simulink library "POSTPROC"  (Simulink 9.0)
settings: Solver=VariableStepAuto  StartTime=0.0  StopTime=10.0  RelTol=1e-3
undefined symbols (not defined in the file or in its folder): DYN_SC_par, SEN_GYR_par, SEN_MTM_par, SEN_SOL_par, SEN_SSS_par, sim_par
libraries: LIB_ROT x24, LIB_ORB x1
settings Model: Creator=alger  LastModifiedBy=alger

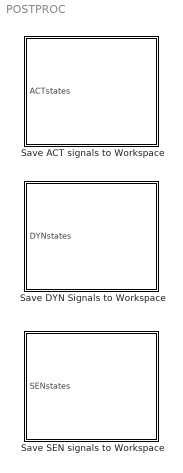
== system POSTPROC ==
  Save ACT signals to Workspace : Subsystem
  Save DYN Signals to Workspace : Subsystem
  Save SEN signals to Workspace : Subsystem

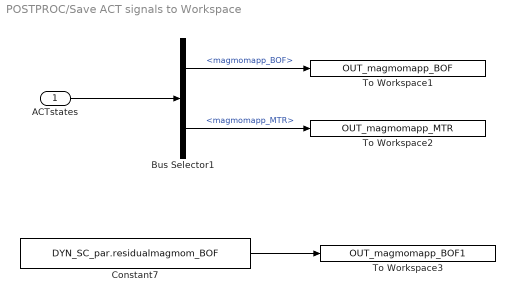
== system POSTPROC/Save ACT signals to Workspace ==
  ACTstates : Inport  SampleTime=sim_par.t_sample
  Bus Selector1 : BusSelector  OutputSignals=magmomapp_BOF,magmomapp_MTR
  Constant7 : Constant  Value=DYN_SC_par.residualmagmom_BOF
  To Workspace1 : ToWorkspace  VariableName=OUT_magmomapp_BOF  SaveFormat=Structure With Time  SampleTime=sim_par.t_sample
  To Workspace2 : ToWorkspace  VariableName=OUT_magmomapp_MTR  SaveFormat=Structure With Time  SampleTime=sim_par.t_sample
  To Workspace3 : ToWorkspace  VariableName=OUT_magmomapp_BOF1  SaveFormat=Structure With Time  SampleTime=sim_par.t_sample
  wires:
  Bus Selector1/2 -> To Workspace2/1  "<magmomapp_MTR>"
  Bus Selector1/1 -> To Workspace1/1  "<magmomapp_BOF>"
  ACTstates/1 -> Bus Selector1/1
  Constant7/1 -> To Workspace3/1

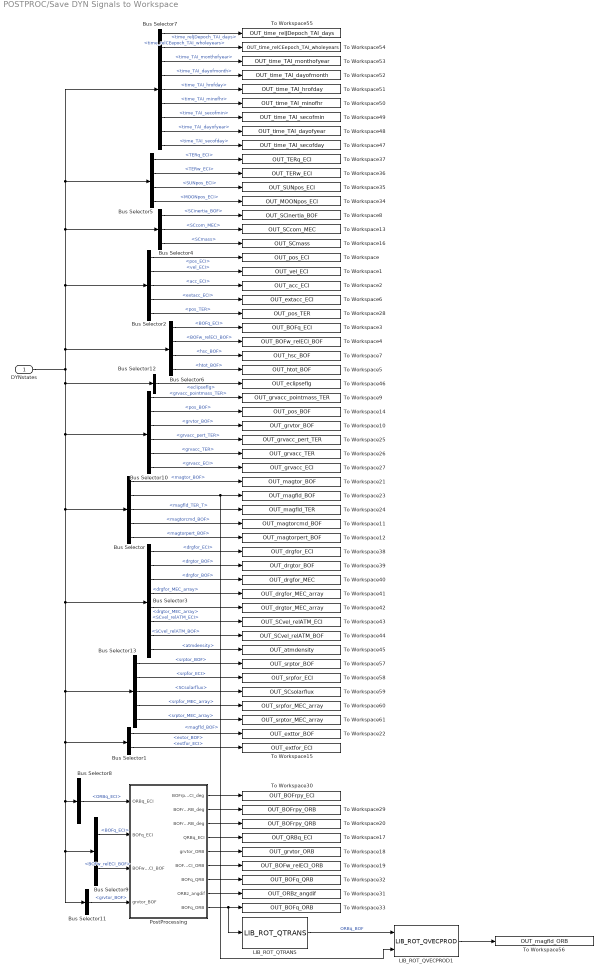
== system POSTPROC/Save DYN Signals to Workspace ==
  DYNstates : Inport  SampleTime=sim_par.t_sample
  Bus Selector : BusSelector  OutputSignals=magtor_BOF,magfld_BOF,magfld_TER_T,magtorcmd_BOF,magtorpert_BOF
  Bus Selector1 : BusSelector  OutputSignals=extor_BOF,extfor_ECI
  Bus Selector10 : BusSelector  OutputSignals=grvacc_pointmass_TER,pos_BOF,grvtor_BOF,grvacc_pert_TER,grvacc_TER,grvacc_ECI
  Bus Selector11 : BusSelector  OutputSignals=grvtor_BOF
  Bus Selector12 : BusSelector  OutputSignals=eclipseflg
  Bus Selector13 : BusSelector  OutputSignals=srptor_BOF,srpfor_ECI,SCsolarflux,srpfor_MEC_array,srptor_MEC_array
  Bus Selector2 : BusSelector  OutputSignals=pos_ECI,vel_ECI,acc_ECI,extacc_ECI,pos_TER
  Bus Selector3 : BusSelector  OutputSignals=drgfor_ECI,drgtor_BOF,drgfor_BOF,drgfor_MEC_array,drgtor_MEC_array,SCvel_relATM_ECI,SCvel_relATM_BOF,atmdensity
  Bus Selector4 : BusSelector  OutputSignals=SCinertia_BOF,SCcom_MEC,SCmass
  Bus Selector5 : BusSelector  OutputSignals=TERq_ECI,TERw_ECI,SUNpos_ECI,MOONpos_ECI
  Bus Selector6 : BusSelector  OutputSignals=BOFq_ECI,BOFw_relECI_BOF,hsc_BOF,htot_BOF
  Bus Selector7 : BusSelector  OutputSignals=time_relJDepoch_TAI_days,time_relCEepoch_TAI_wholeyears,time_TAI_monthofyear,time_TAI_dayofmonth,time_TAI_hrofday,time_TAI_minofhr,time_TAI_secofmin,time_TAI_dayofyear,time_TAI_secofday
  Bus Selector8 : BusSelector  OutputSignals=ORBq_ECI
  Bus Selector9 : BusSelector  OutputSignals=BOFq_ECI,BOFw_relECI_BOF
  LIB_ROT_QTRANS : LIB_ROT/LIB_ROT_QTRANS
  LIB_ROT_QVECPROD1 : LIB_ROT/LIB_ROT_QVECPROD
  PostProcessing : Subsystem
  To Workspace : ToWorkspace  VariableName=OUT_pos_ECI  SaveFormat=Structure With Time  SampleTime=sim_par.t_sample
  To Workspace1 : ToWorkspace  VariableName=OUT_vel_ECI  SaveFormat=Structure With Time  SampleTime=sim_par.t_sample
  To Workspace10 : ToWorkspace  VariableName=OUT_grvtor_BOF  SaveFormat=Structure With Time  SampleTime=sim_par.t_sample
  To Workspace11 : ToWorkspace  VariableName=OUT_magtorcmd_BOF  SaveFormat=Structure With Time  SampleTime=sim_par.t_sample
  To Workspace12 : ToWorkspace  VariableName=OUT_magtorpert_BOF  SaveFormat=Structure With Time  SampleTime=sim_par.t_sample
  To Workspace13 : ToWorkspace  VariableName=OUT_SCcom_MEC  SaveFormat=Structure With Time  SampleTime=sim_par.t_sample
  To Workspace14 : ToWorkspace  VariableName=OUT_pos_BOF  SaveFormat=Structure With Time  SampleTime=sim_par.t_sample
  To Workspace15 : ToWorkspace  VariableName=OUT_extfor_ECI  SaveFormat=Structure With Time  SampleTime=sim_par.t_sample
  To Workspace16 : ToWorkspace  VariableName=OUT_SCmass  SaveFormat=Structure With Time  SampleTime=sim_par.t_sample
  To Workspace17 : ToWorkspace  VariableName=OUT_QRBq_ECI  SaveFormat=Structure With Time  SampleTime=sim_par.t_sample
  To Workspace18 : ToWorkspace  VariableName=OUT_grvtor_ORB  SaveFormat=Structure With Time  SampleTime=sim_par.t_sample
  To Workspace19 : ToWorkspace  VariableName=OUT_BOFw_relECI_ORB  SaveFormat=Structure With Time  SampleTime=sim_par.t_sample
  To Workspace2 : ToWorkspace  VariableName=OUT_acc_ECI  SaveFormat=Structure With Time  SampleTime=sim_par.t_sample
  To Workspace20 : ToWorkspace  VariableName=OUT_BOFrpy_QRB  SaveFormat=Structure With Time  SampleTime=sim_par.t_sample
  To Workspace21 : ToWorkspace  VariableName=OUT_magtor_BOF  SaveFormat=Structure With Time  SampleTime=sim_par.t_sample
  To Workspace22 : ToWorkspace  VariableName=OUT_exttor_BOF  SaveFormat=Structure With Time  SampleTime=sim_par.t_sample
  To Workspace23 : ToWorkspace  VariableName=OUT_magfld_BOF  SaveFormat=Structure With Time  SampleTime=sim_par.t_sample
  To Workspace24 : ToWorkspace  VariableName=OUT_magfld_TER  SaveFormat=Structure With Time  SampleTime=sim_par.t_sample
  To Workspace25 : ToWorkspace  VariableName=OUT_grvacc_pert_TER  SaveFormat=Structure With Time  SampleTime=sim_par.t_sample
  To Workspace26 : ToWorkspace  VariableName=OUT_grvacc_TER  SaveFormat=Structure With Time  SampleTime=sim_par.t_sample
  To Workspace27 : ToWorkspace  VariableName=OUT_grvacc_ECI  SaveFormat=Structure With Time  SampleTime=sim_par.t_sample
  To Workspace28 : ToWorkspace  VariableName=OUT_pos_TER  SaveFormat=Structure With Time  SampleTime=sim_par.t_sample
  To Workspace29 : ToWorkspace  VariableName=OUT_BOFrpy_ORB  SaveFormat=Structure With Time  SampleTime=sim_par.t_sample
  To Workspace3 : ToWorkspace  VariableName=OUT_BOFq_ECI  SaveFormat=Structure With Time  SampleTime=sim_par.t_sample
  To Workspace30 : ToWorkspace  VariableName=OUT_BOFrpy_ECI  SaveFormat=Structure With Time  SampleTime=sim_par.t_sample
  To Workspace31 : ToWorkspace  VariableName=OUT_ORBz_angdif  SaveFormat=Structure With Time  SampleTime=sim_par.t_sample
  To Workspace32 : ToWorkspace  VariableName=OUT_BOFq_QRB  SaveFormat=Structure With Time  SampleTime=sim_par.t_sample
  To Workspace33 : ToWorkspace  VariableName=OUT_BOFq_ORB  SaveFormat=Structure With Time  SampleTime=sim_par.t_sample
  To Workspace34 : ToWorkspace  VariableName=OUT_MOONpos_ECI  SaveFormat=Structure With Time  SampleTime=sim_par.t_sample
  To Workspace35 : ToWorkspace  VariableName=OUT_SUNpos_ECI  SaveFormat=Structure With Time  SampleTime=sim_par.t_sample
  To Workspace36 : ToWorkspace  VariableName=OUT_TERw_ECI  SaveFormat=Structure With Time  SampleTime=sim_par.t_sample
  To Workspace37 : ToWorkspace  VariableName=OUT_TERq_ECI  SaveFormat=Structure With Time  SampleTime=sim_par.t_sample
  To Workspace38 : ToWorkspace  VariableName=OUT_drgfor_ECI  SaveFormat=Structure With Time  SampleTime=sim_par.t_sample
  To Workspace39 : ToWorkspace  VariableName=OUT_drgtor_BOF  SaveFormat=Structure With Time  SampleTime=sim_par.t_sample
  To Workspace4 : ToWorkspace  VariableName=OUT_BOFw_relECI_BOF  SaveFormat=Structure With Time  SampleTime=sim_par.t_sample
  To Workspace40 : ToWorkspace  VariableName=OUT_drgfor_MEC  SaveFormat=Structure With Time  SampleTime=sim_par.t_sample
  To Workspace41 : ToWorkspace  VariableName=OUT_drgfor_MEC_array  SaveFormat=Structure With Time  SampleTime=sim_par.t_sample
  To Workspace42 : ToWorkspace  VariableName=OUT_drgtor_MEC_array  SaveFormat=Structure With Time  SampleTime=sim_par.t_sample
  To Workspace43 : ToWorkspace  VariableName=OUT_SCvel_relATM_ECI  SaveFormat=Structure With Time  SampleTime=sim_par.t_sample
  To Workspace44 : ToWorkspace  VariableName=OUT_SCvel_relATM_BOF  SaveFormat=Structure With Time  SampleTime=sim_par.t_sample
  To Workspace45 : ToWorkspace  VariableName=OUT_atmdensity  SaveFormat=Structure With Time  SampleTime=sim_par.t_sample
  To Workspace46 : ToWorkspace  VariableName=OUT_eclipseflg  SaveFormat=Structure With Time  SampleTime=sim_par.t_sample
  To Workspace47 : ToWorkspace  VariableName=OUT_time_TAI_secofday  SaveFormat=Structure With Time  SampleTime=sim_par.t_sample
  To Workspace48 : ToWorkspace  VariableName=OUT_time_TAI_dayofyear  SaveFormat=Structure With Time  SampleTime=sim_par.t_sample
  To Workspace49 : ToWorkspace  VariableName=OUT_time_TAI_secofmin  SaveFormat=Structure With Time  SampleTime=sim_par.t_sample
  To Workspace5 : ToWorkspace  VariableName=OUT_htot_BOF  SaveFormat=Structure With Time  SampleTime=sim_par.t_sample
  To Workspace50 : ToWorkspace  VariableName=OUT_time_TAI_minofhr  SaveFormat=Structure With Time  SampleTime=sim_par.t_sample
  To Workspace51 : ToWorkspace  VariableName=OUT_time_TAI_hrofday  SaveFormat=Structure With Time  SampleTime=sim_par.t_sample
  To Workspace52 : ToWorkspace  VariableName=OUT_time_TAI_dayofmonth  SaveFormat=Structure With Time  SampleTime=sim_par.t_sample
  To Workspace53 : ToWorkspace  VariableName=OUT_time_TAI_monthofyear  SaveFormat=Structure With Time  SampleTime=sim_par.t_sample
  To Workspace54 : ToWorkspace  VariableName=OUT_time_relCEepoch_TAI_wholeyears  SaveFormat=Structure With Time  SampleTime=sim_par.t_sample
  To Workspace55 : ToWorkspace  VariableName=OUT_time_relJDepoch_TAI_days  SaveFormat=Structure With Time  SampleTime=sim_par.t_sample
  To Workspace56 : ToWorkspace  VariableName=OUT_magfld_ORB  SaveFormat=Structure With Time  SampleTime=sim_par.t_sample
  To Workspace57 : ToWorkspace  VariableName=OUT_srptor_BOF  SaveFormat=Structure With Time  SampleTime=sim_par.t_sample
  To Workspace58 : ToWorkspace  VariableName=OUT_srpfor_ECI  SaveFormat=Structure With Time  SampleTime=sim_par.t_sample
  To Workspace59 : ToWorkspace  VariableName=OUT_SCsolarflux  SaveFormat=Structure With Time  SampleTime=sim_par.t_sample
  To Workspace6 : ToWorkspace  VariableName=OUT_extacc_ECI  SaveFormat=Structure With Time  SampleTime=sim_par.t_sample
  To Workspace60 : ToWorkspace  VariableName=OUT_srpfor_MEC_array  SaveFormat=Structure With Time  SampleTime=sim_par.t_sample
  To Workspace61 : ToWorkspace  VariableName=OUT_srptor_MEC_array  SaveFormat=Structure With Time  SampleTime=sim_par.t_sample
  To Workspace7 : ToWorkspace  VariableName=OUT_hsc_BOF  SaveFormat=Structure With Time  SampleTime=sim_par.t_sample
  To Workspace8 : ToWorkspace  VariableName=OUT_SCinertia_BOF  SaveFormat=Structure With Time  SampleTime=sim_par.t_sample
  To Workspace9 : ToWorkspace  VariableName=OUT_grvacc_pointmass_TER  SaveFormat=Structure With Time  SampleTime=sim_par.t_sample
  wires:
  Bus Selector13/5 -> To Workspace61/1  "<srptor_MEC_array>"
  Bus Selector13/4 -> To Workspace60/1  "<srpfor_MEC_array>"
  Bus Selector13/3 -> To Workspace59/1  "<SCsolarflux>"
  Bus Selector13/2 -> To Workspace58/1  "<srpfor_ECI>"
  Bus Selector13/1 -> To Workspace57/1  "<srptor_BOF>"
  LIB_ROT_QVECPROD1/1 -> To Workspace56/1
  LIB_ROT_QTRANS/1 -> LIB_ROT_QVECPROD1/1  "ORBq_BOF"
  Bus Selector/2 -> LIB_ROT_QVECPROD1/2, To Workspace23/1  "<magfld_BOF>"
  Bus Selector10/2 -> To Workspace14/1  "<pos_BOF>"
  Bus Selector6/4 -> To Workspace5/1  "<htot_BOF>"
  Bus Selector2/3 -> To Workspace2/1  "<acc_ECI>"
  Bus Selector4/3 -> To Workspace16/1  "<SCmass>"
  Bus Selector5/4 -> To Workspace34/1  "<MOONpos_ECI>"
  Bus Selector6/1 -> To Workspace3/1  "<BOFq_ECI>"
  Bus Selector2/5 -> To Workspace28/1  "<pos_TER>"
  Bus Selector2/2 -> To Workspace1/1  "<vel_ECI>"
  Bus Selector5/2 -> To Workspace36/1  "<TERw_ECI>"
  Bus Selector3/2 -> To Workspace39/1  "<drgtor_BOF>"
  Bus Selector3/3 -> To Workspace40/1  "<drgfor_BOF>"
  Bus Selector4/2 -> To Workspace13/1  "<SCcom_MEC>"
  Bus Selector4/1 -> To Workspace8/1  "<SCinertia_BOF>"
  Bus Selector3/4 -> To Workspace41/1  "<drgfor_MEC_array>"
  Bus Selector3/5 -> To Workspace42/1  "<drgtor_MEC_array>"
  Bus Selector/5 -> To Workspace12/1  "<magtorpert_BOF>"
  Bus Selector/4 -> To Workspace11/1  "<magtorcmd_BOF>"
  Bus Selector2/4 -> To Workspace6/1  "<extacc_ECI>"
  Bus Selector/3 -> To Workspace24/1  "<magfld_TER_T>"
  Bus Selector6/3 -> To Workspace7/1  "<hsc_BOF>"
  Bus Selector6/2 -> To Workspace4/1  "<BOFw_relECI_BOF>"
  Bus Selector5/3 -> To Workspace35/1  "<SUNpos_ECI>"
  Bus Selector10/4 -> To Workspace25/1  "<grvacc_pert_TER>"
  Bus Selector2/1 -> To Workspace/1  "<pos_ECI>"
  Bus Selector10/3 -> To Workspace10/1  "<grvtor_BOF>"
  Bus Selector/1 -> To Workspace21/1  "<magtor_BOF>"
  Bus Selector10/6 -> To Workspace27/1  "<grvacc_ECI>"
  Bus Selector10/1 -> To Workspace9/1  "<grvacc_pointmass_TER>"
  Bus Selector10/5 -> To Workspace26/1  "<grvacc_TER>"
  Bus Selector5/1 -> To Workspace37/1  "<TERq_ECI>"
  PostProcessing/9(BOFq_ORB) -> To Workspace33/1, LIB_ROT_QTRANS/1
  Bus Selector12/1 -> To Workspace46/1  "<eclipseflg>"
  Bus Selector9/1 -> PostProcessing/2(BOFq_ECI)  "<BOFq_ECI>"
  PostProcessing/5(grvtor_ORB) -> To Workspace18/1
  Bus Selector9/2 -> PostProcessing/3(BOFw_relECI_BOF)  "<BOFw_relECI_BOF>"
  PostProcessing/6(BOFw_relECI_ORB) -> To Workspace19/1
  PostProcessing/4(QRBq_ECI) -> To Workspace17/1
  Bus Selector1/2 -> To Workspace15/1  "<extfor_ECI>"
  Bus Selector3/1 -> To Workspace38/1  "<drgfor_ECI>"
  Bus Selector7/3 -> To Workspace53/1  "<time_TAI_monthofyear>"
  PostProcessing/1(BOFrpy_ECI_deg) -> To Workspace30/1
  Bus Selector7/1 -> To Workspace55/1  "<time_relJDepoch_TAI_days>"
  PostProcessing/7(BOFq_QRB) -> To Workspace32/1
  Bus Selector7/9 -> To Workspace47/1  "<time_TAI_secofday>"
  Bus Selector7/8 -> To Workspace48/1  "<time_TAI_dayofyear>"
  PostProcessing/8(ORBz_angdif) -> To Workspace31/1
  Bus Selector7/2 -> To Workspace54/1  "<time_relCEepoch_TAI_wholeyears>"
  Bus Selector7/7 -> To Workspace49/1  "<time_TAI_secofmin>"
  Bus Selector7/5 -> To Workspace51/1  "<time_TAI_hrofday>"
  Bus Selector7/6 -> To Workspace50/1  "<time_TAI_minofhr>"
  Bus Selector7/4 -> To Workspace52/1  "<time_TAI_dayofmonth>"
  DYNstates/1 -> Bus Selector2/1, Bus Selector7/1, Bus Selector5/1, Bus Selector4/1, Bus Selector6/1, Bus Selector10/1, Bus Selector/1, Bus Selector3/1, Bus Selector13/1, Bus Selector1/1, Bus Selector8/1, Bus Selector9/1, Bus Selector11/1, Bus Selector12/1
  PostProcessing/2(BOFrpy_ORB_deg) -> To Workspace29/1
  PostProcessing/3(BOFrpy_QRB_deg) -> To Workspace20/1
  Bus Selector8/1 -> PostProcessing/1(ORBq_ECI)  "<ORBq_ECI>"
  Bus Selector11/1 -> PostProcessing/4(grvtor_BOF)  "<grvtor_BOF>"
  Bus Selector3/6 -> To Workspace43/1  "<SCvel_relATM_ECI>"
  Bus Selector3/8 -> To Workspace45/1  "<atmdensity>"
  Bus Selector3/7 -> To Workspace44/1  "<SCvel_relATM_BOF>"
  Bus Selector1/1 -> To Workspace22/1  "<extor_BOF>"

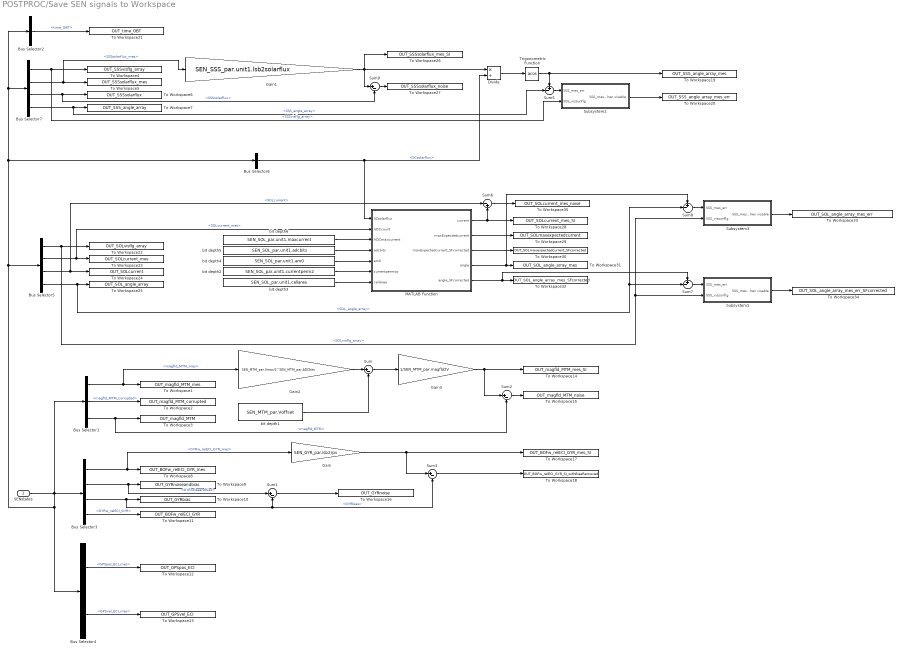
== system POSTPROC/Save SEN signals to Workspace ==
  SENstates : Inport  SampleTime=sim_par.t_sample
  Bus Selector1 : BusSelector  OutputSignals=magfld_MTM_mes,magfld_MTM_corrupted,magfld_MTM
  Bus Selector2 : BusSelector  OutputSignals=time_OBT
  Bus Selector3 : BusSelector  OutputSignals=GYRw_relECI_GYR_mes,GYRnoiseandbias,GYRbias,GYRw_relECI_GYR
  Bus Selector4 : BusSelector  OutputSignals=GPSpos_ECI_mes,GPSvel_ECI_mes
  Bus Selector5 : BusSelector  OutputSignals=SOLvisflg_array,SOLcurrent_mes,SOLcurrent,SOL_angle_array
  Bus Selector6 : BusSelector  OutputSignals=SCsolarflux
  Bus Selector7 : BusSelector  OutputSignals=SSSvisflg_array,SSSsolarflux_mes,SSSsolarflux,SSS_angle_array
  Divide : Product  Inputs=*/
  Gain : Gain  Gain=SEN_GYR_par.lsb2rps
  Gain1 : Gain  Gain=SEN_SSS_par.unit1.lsb2solarflux
  Gain2 : Gain  Gain=SEN_MTM_par.Vmax/2^SEN_MTM_par.ADCbits
  Gain3 : Gain  Gain=1/SEN_MTM_par.magfld2V
  MATLAB Function : MATLAB Function  TreatAsAtomicUnit=on
  Subsystem1 : Subsystem
  Subsystem2 : Subsystem
  Subsystem3 : Subsystem
  Sum{,1..3,9} (5 alike) : Sum  Inputs=|+-
  Sum5 : Sum  Inputs=+-|
  Sum6 : Sum  Inputs=|-+
  Sum7 : Sum  Inputs=+-|
  Sum8 : Sum  Inputs=+-|
  To Workspace1 : ToWorkspace  VariableName=OUT_magfld_MTM_mes  SaveFormat=Structure With Time  SampleTime=sim_par.t_sample
  To Workspace10 : ToWorkspace  VariableName=OUT_GYRbias  SaveFormat=Structure With Time  SampleTime=sim_par.t_sample
  To Workspace11 : ToWorkspace  VariableName=OUT_BOFw_relECI_GYR  SaveFormat=Structure With Time  SampleTime=sim_par.t_sample
  To Workspace12 : ToWorkspace  VariableName=OUT_GPSpos_ECI  SaveFormat=Structure With Time  SampleTime=sim_par.t_sample
  To Workspace13 : ToWorkspace  VariableName=OUT_GPSvel_ECI  SaveFormat=Structure With Time  SampleTime=sim_par.t_sample
  To Workspace14 : ToWorkspace  VariableName=OUT_magfld_MTM_mes_SI  SaveFormat=Structure With Time  SampleTime=sim_par.t_sample
  To Workspace15 : ToWorkspace  VariableName=OUT_magfld_MTM_noise  SaveFormat=Structure With Time  SampleTime=sim_par.t_sample
  To Workspace16 : ToWorkspace  VariableName=OUT_GYRnoise  SaveFormat=Structure With Time  SampleTime=sim_par.t_sample
  To Workspace17 : ToWorkspace  VariableName=OUT_BOFw_relECI_GYR_mes_SI  SaveFormat=Structure With Time  SampleTime=sim_par.t_sample
  To Workspace18 : ToWorkspace  VariableName=OUT_BOFw_relECI_GYR_SI_withBiasRemoved  SaveFormat=Structure With Time  SampleTime=sim_par.t_sample
  To Workspace19 : ToWorkspace  VariableName=OUT_SSS_angle_array_mes  SaveFormat=Structure With Time  SampleTime=sim_par.t_sample
  To Workspace2 : ToWorkspace  VariableName=OUT_magfld_MTM_corrupted  SaveFormat=Structure With Time  SampleTime=sim_par.t_sample
  To Workspace20 : ToWorkspace  VariableName=OUT_SSS_angle_array_mes_err  SaveFormat=Structure With Time  SampleTime=sim_par.t_sample
  To Workspace21 : ToWorkspace  VariableName=OUT_time_OBT  SaveFormat=Structure With Time  SampleTime=sim_par.t_sample
  To Workspace22 : ToWorkspace  VariableName=OUT_SOLvisflg_array  SaveFormat=Structure With Time  SampleTime=sim_par.t_sample
  To Workspace23 : ToWorkspace  VariableName=OUT_SOLcurrent_mes  SaveFormat=Structure With Time  SampleTime=sim_par.t_sample
  To Workspace24 : ToWorkspace  VariableName=OUT_SOLcurrent  SaveFormat=Structure With Time  SampleTime=sim_par.t_sample
  To Workspace25 : ToWorkspace  VariableName=OUT_SOL_angle_array  SaveFormat=Structure With Time  SampleTime=sim_par.t_sample
  To Workspace26 : ToWorkspace  VariableName=OUT_SSSsolarflux_mes_SI  SaveFormat=Structure With Time  SampleTime=sim_par.t_sample
  To Workspace27 : ToWorkspace  VariableName=OUT_SSSsolarflux_noise  SaveFormat=Structure With Time  SampleTime=sim_par.t_sample
  To Workspace28 : ToWorkspace  VariableName=OUT_SOLcurrent_mes_SI  SaveFormat=Structure With Time  SampleTime=sim_par.t_sample
  To Workspace29 : ToWorkspace  VariableName=OUT_SOLmaxexpectedcurrent  SaveFormat=Structure With Time  SampleTime=sim_par.t_sample
  To Workspace3 : ToWorkspace  VariableName=OUT_magfld_MTM  SaveFormat=Structure With Time  SampleTime=sim_par.t_sample
  To Workspace30 : ToWorkspace  VariableName=OUT_SOLmaxexpectedcurrent_SFcorrected  SaveFormat=Structure With Time  SampleTime=sim_par.t_sample
  To Workspace31 : ToWorkspace  VariableName=OUT_SOL_angle_array_mes  SaveFormat=Structure With Time  SampleTime=sim_par.t_sample
  To Workspace32 : ToWorkspace  VariableName=OUT_SOL_angle_array_mes_SFcorrected  SaveFormat=Structure With Time  SampleTime=sim_par.t_sample
  To Workspace33 : ToWorkspace  VariableName=OUT_SOL_angle_array_mes_err  SaveFormat=Structure With Time  SampleTime=sim_par.t_sample
  To Workspace34 : ToWorkspace  VariableName=OUT_SOL_angle_array_mes_err_SFcorrected  SaveFormat=Structure With Time  SampleTime=sim_par.t_sample
  To Workspace35 : ToWorkspace  VariableName=OUT_SOLcurrent_mes_noise  SaveFormat=Structure With Time  SampleTime=sim_par.t_sample
  To Workspace4 : ToWorkspace  VariableName=OUT_SSSvisflg_array  SaveFormat=Structure With Time  SampleTime=sim_par.t_sample
  To Workspace5 : ToWorkspace  VariableName=OUT_SSSsolarflux_mes  SaveFormat=Structure With Time  SampleTime=sim_par.t_sample
  To Workspace6 : ToWorkspace  VariableName=OUT_SSSsolarflux  SaveFormat=Structure With Time  SampleTime=sim_par.t_sample
  To Workspace7 : ToWorkspace  VariableName=OUT_SSS_angle_array  SaveFormat=Structure With Time  SampleTime=sim_par.t_sample
  To Workspace8 : ToWorkspace  VariableName=OUT_BOFw_relECI_GYR_mes  SaveFormat=Structure With Time  SampleTime=sim_par.t_sample
  To Workspace9 : ToWorkspace  VariableName=OUT_GYRnoiseandbias  SaveFormat=Structure With Time  SampleTime=sim_par.t_sample
  Trigonometric Function : Trigonometry  Operator=acos  OutputSignalType=real
  bit depth1 : Constant  Value=SEN_MTM_par.Voffset
  bit depth2 : Constant  Value=SEN_SOL_par.unit1.currentperm2
  bit depth3 : Constant  Value=SEN_SOL_par.unit1.cellarea
  bit depth4 : Constant  Value=SEN_SOL_par.unit1.am0
  bit depth5 : Constant  Value=SEN_SOL_par.unit1.adcbits
  bit depth6 : Constant  Value=SEN_SOL_par.unit1.maxcurrent
  wires:
  MATLAB Function/3(maxExpectedcurrent_SFcorrected) -> To Workspace30/1
  Sum9/1 -> To Workspace27/1
  Divide/1 -> Trigonometric Function/1
  MATLAB Function/2(maxExpectedcurrent) -> To Workspace29/1
  Subsystem3/1(SSS_mes_err when visable) -> To Workspace33/1
  Sum8/1 -> Subsystem3/1(SSS_mes_err)
  MATLAB Function/4(angle) -> Sum8/1, To Workspace31/1
  Bus Selector5/4 -> To Workspace25/1, Sum8/2, Sum7/2  "<SOL_angle_array>"
  Bus Selector5/1 -> To Workspace22/1, Subsystem3/2(SSS_vissunflg), Subsystem1/2(SSS_vissunflg)  "<SOLvisflg_array>"
  Subsystem1/1(SSS_mes_err when visable) -> To Workspace34/1
  Sum7/1 -> Subsystem1/1(SSS_mes_err)
  MATLAB Function/5(angle_SFcorrected) -> To Workspace32/1, Sum7/1
  Sum6/1 -> To Workspace35/1
  bit depth6/1 -> MATLAB Function/3(ADCmaxcurrent)
  bit depth5/1 -> MATLAB Function/4(adcbits)
  bit depth4/1 -> MATLAB Function/5(am0)
  bit depth3/1 -> MATLAB Function/7(cellarea)
  bit depth2/1 -> MATLAB Function/6(currentpermsq)
  MATLAB Function/1(current) -> Sum6/2, To Workspace28/1
  Bus Selector6/1 -> MATLAB Function/1(SCsolarflux), Divide/2  "<SCsolarflux>"
  Bus Selector5/3 -> To Workspace24/1, Sum6/1  "<SOLcurrent>"
  Bus Selector5/2 -> To Workspace23/1, MATLAB Function/2(ADCcount)  "<SOLcurrent_mes>"
  Bus Selector2/1 -> To Workspace21/1  "<time_OBT>"
  SENstates/1 -> Bus Selector5/1, Bus Selector6/1, Bus Selector7/1, Bus Selector2/1, Bus Selector4/1, Bus Selector1/1, Bus Selector3/1
  Bus Selector1/1 -> Gain2/1, To Workspace1/1  "<magfld_MTM_mes>"
  Bus Selector1/2 -> To Workspace2/1  "<magfld_MTM_corrupted>"
  Bus Selector1/3 -> Sum2/2, To Workspace3/1  "<magfld_MTM>"
  Bus Selector7/1 -> To Workspace4/1, Subsystem2/2(SSS_vissunflg)  "<SSSvisflg_array>"
  Bus Selector7/4 -> Sum5/2, To Workspace7/1  "<SSS_angle_array>"
  Bus Selector7/3 -> To Workspace6/1, Sum9/2  "<SSSsolarflux>"
  Bus Selector7/2 -> Gain1/1, To Workspace5/1  "<SSSsolarflux_mes>"
  Bus Selector3/1 -> Gain/1, To Workspace8/1  "<GYRw_relECI_GYR_mes>"
  Bus Selector3/2 -> Sum1/1, To Workspace9/1  "<GYRnoiseandbias>"
  Bus Selector3/3 -> Sum1/2, Sum3/2, To Workspace10/1  "<GYRbias>"
  Bus Selector3/4 -> To Workspace11/1  "<GYRw_relECI_GYR>"
  Bus Selector4/1 -> To Workspace12/1  "<GPSpos_ECI_mes>"
  Bus Selector4/2 -> To Workspace13/1  "<GPSvel_ECI_mes>"
  Sum/1 -> Gain3/1
  Gain2/1 -> Sum/1
  bit depth1/1 -> Sum/2
  Gain3/1 -> Sum2/1, To Workspace14/1
  Sum2/1 -> To Workspace15/1
  Sum1/1 -> To Workspace16/1
  Gain/1 -> Sum3/1, To Workspace17/1
  Sum3/1 -> To Workspace18/1
  Gain1/1 -> Sum9/1, Divide/1, To Workspace26/1
  Sum5/1 -> Subsystem2/1(SSS_mes_err)
  Trigonometric Function/1 -> To Workspace19/1, Sum5/1
  Subsystem2/1(SSS_mes_err when visable) -> To Workspace20/1

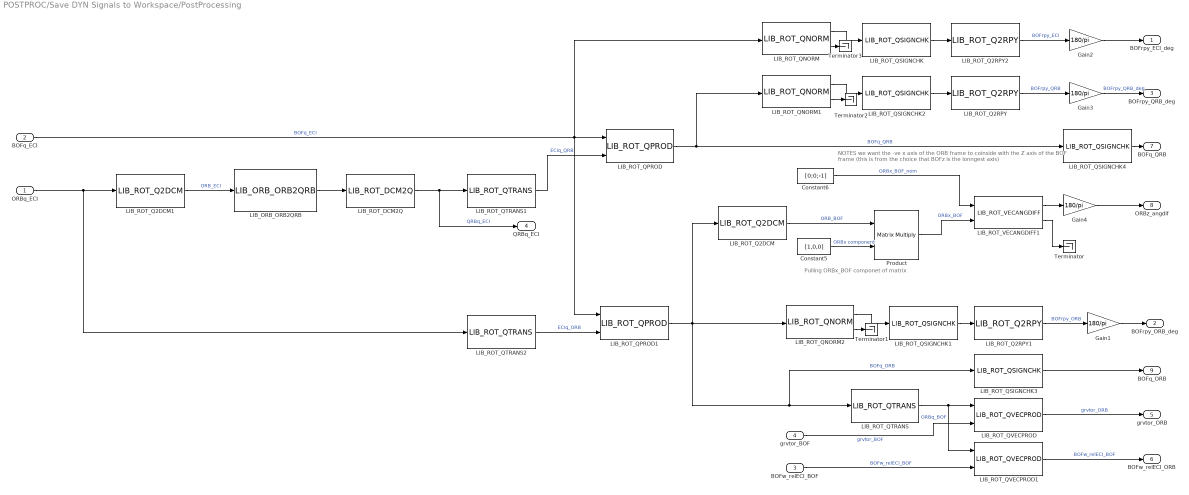
== system POSTPROC/Save DYN Signals to Workspace/PostProcessing ==
  note: Pulling ORBx_BOF componet of matrix
  note: NOTES
      | we want the -ve x axis of the ORB frame to coinside with the Z axis of the BOF frame
      | (this is from the choice that BOFz is the lonngest axis)
  ORBq_ECI : Inport
  BOFq_ECI : Inport  Port=2
  BOFw_relECI_BOF : Inport  Port=3
  grvtor_BOF : Inport  Port=4
  Constant5 : Constant  Value=[1,0,0]
  Constant6 : Constant  Value=[0;0;-1]
  Gain{1..4} (4 alike) : Gain  Gain=180/pi
  LIB_ORB_ORB2QRB : LIB_ORB/LIB_ORB_ORB2QRB
  LIB_ROT_DCM2Q : LIB_ROT/LIB_ROT_DCM2Q
  LIB_ROT_Q2DCM : LIB_ROT/LIB_ROT_Q2DCM
  LIB_ROT_Q2DCM1 : LIB_ROT/LIB_ROT_Q2DCM
  LIB_ROT_Q2RPY : LIB_ROT/LIB_ROT_Q2RPY
  LIB_ROT_Q2RPY1 : LIB_ROT/LIB_ROT_Q2RPY
  LIB_ROT_Q2RPY2 : LIB_ROT/LIB_ROT_Q2RPY
  LIB_ROT_QNORM : LIB_ROT/LIB_ROT_QNORM  zero_tol=0
  LIB_ROT_QNORM1 : LIB_ROT/LIB_ROT_QNORM  zero_tol=0
  LIB_ROT_QNORM2 : LIB_ROT/LIB_ROT_QNORM  zero_tol=0
  LIB_ROT_QPROD : LIB_ROT/LIB_ROT_QPROD
  LIB_ROT_QPROD1 : LIB_ROT/LIB_ROT_QPROD
  LIB_ROT_QSIGNCHK{,1..4} (5 alike) : LIB_ROT/LIB_ROT_QSIGNCHK
  LIB_ROT_QTRANS : LIB_ROT/LIB_ROT_QTRANS
  LIB_ROT_QTRANS1 : LIB_ROT/LIB_ROT_QTRANS
  LIB_ROT_QTRANS2 : LIB_ROT/LIB_ROT_QTRANS
  LIB_ROT_QVECPROD : LIB_ROT/LIB_ROT_QVECPROD
  LIB_ROT_QVECPROD1 : LIB_ROT/LIB_ROT_QVECPROD
  LIB_ROT_VECANGDIFF1 : LIB_ROT/LIB_ROT_VECANGDIFF  zero_tol=0
  Product : Product  Multiplication=Matrix(*)
  Terminator{,1..3} (4 alike) : Terminator
  BOFrpy_ECI_deg : Outport
  BOFrpy_ORB_deg : Outport  Port=2
  BOFrpy_QRB_deg : Outport  Port=3
  QRBq_ECI : Outport  Port=4
  grvtor_ORB : Outport  Port=5
  BOFw_relECI_ORB : Outport  Port=6
  BOFq_QRB : Outport  Port=7
  ORBz_angdif : Outport  Port=8
  BOFq_ORB : Outport  Port=9
  wires:
  LIB_ROT_QNORM/2 -> Terminator3/1
  LIB_ROT_QNORM1/2 -> Terminator2/1
  LIB_ROT_QNORM2/2 -> Terminator1/1
  LIB_ROT_QNORM/1 -> LIB_ROT_QSIGNCHK/1
  LIB_ROT_QNORM1/1 -> LIB_ROT_QSIGNCHK2/1
  LIB_ROT_QNORM2/1 -> LIB_ROT_QSIGNCHK1/1
  LIB_ROT_QSIGNCHK4/1 -> BOFq_QRB/1
  LIB_ROT_QSIGNCHK3/1 -> BOFq_ORB/1
  LIB_ROT_VECANGDIFF1/1 -> Gain4/1
  Gain4/1 -> ORBz_angdif/1
  LIB_ROT_QPROD1/1 -> LIB_ROT_Q2DCM/1, LIB_ROT_QNORM2/1, LIB_ROT_QTRANS/1, LIB_ROT_QSIGNCHK3/1  "BOFq_ORB"
  LIB_ROT_QTRANS/1 -> LIB_ROT_QVECPROD1/1, LIB_ROT_QVECPROD/1  "ORBq_BOF"
  LIB_ROT_QVECPROD/1 -> grvtor_ORB/1  "grvtor_ORB"
  LIB_ROT_QVECPROD1/1 -> BOFw_relECI_ORB/1  "BOFw_relECI_BOF"
  LIB_ROT_QSIGNCHK1/1 -> LIB_ROT_Q2RPY1/1
  LIB_ROT_Q2RPY1/1 -> Gain1/1  "BOFrpy_ORB"
  LIB_ROT_QSIGNCHK/1 -> LIB_ROT_Q2RPY2/1
  LIB_ROT_Q2RPY/1 -> Gain3/1  "BOFrpy_QRB"
  LIB_ROT_Q2RPY2/1 -> Gain2/1  "BOFrpy_ECI"
  LIB_ROT_QSIGNCHK2/1 -> LIB_ROT_Q2RPY/1
  LIB_ROT_Q2DCM/1 -> Product/1  "ORB_BOF"
  Constant6/1 -> LIB_ROT_VECANGDIFF1/1  "ORBx_BOF_nom"
  Constant5/1 -> Product/2  "ORBx component"
  Product/1 -> LIB_ROT_VECANGDIFF1/2  "ORBx_BOF"
  grvtor_BOF/1 -> LIB_ROT_QVECPROD/2  "grvtor_BOF"
  BOFw_relECI_BOF/1 -> LIB_ROT_QVECPROD1/2  "BOFw_relECI_BOF"
  LIB_ROT_VECANGDIFF1/2 -> Terminator/1
  Gain2/1 -> BOFrpy_ECI_deg/1
  Gain1/1 -> BOFrpy_ORB_deg/1
  Gain3/1 -> BOFrpy_QRB_deg/1  "BOFrpy_QRB_deg"
  BOFq_ECI/1 -> LIB_ROT_QPROD1/1, LIB_ROT_QPROD/1, LIB_ROT_QNORM/1  "BOFq_ECI"
  LIB_ORB_ORB2QRB/1 -> LIB_ROT_DCM2Q/1
  LIB_ROT_QPROD/1 -> LIB_ROT_QSIGNCHK4/1, LIB_ROT_QNORM1/1  "BOFq_QRB"
  LIB_ROT_DCM2Q/1 -> QRBq_ECI/1, LIB_ROT_QTRANS1/1  "QRBq_ECI"
  LIB_ROT_QTRANS1/1 -> LIB_ROT_QPROD/2  "ECIq_QRB"
  LIB_ROT_Q2DCM1/1 -> LIB_ORB_ORB2QRB/1  "ORB_ECI"
  LIB_ROT_QTRANS2/1 -> LIB_ROT_QPROD1/2  "ECIq_ORB"
  ORBq_ECI/1 -> LIB_ROT_Q2DCM1/1, LIB_ROT_QTRANS2/1

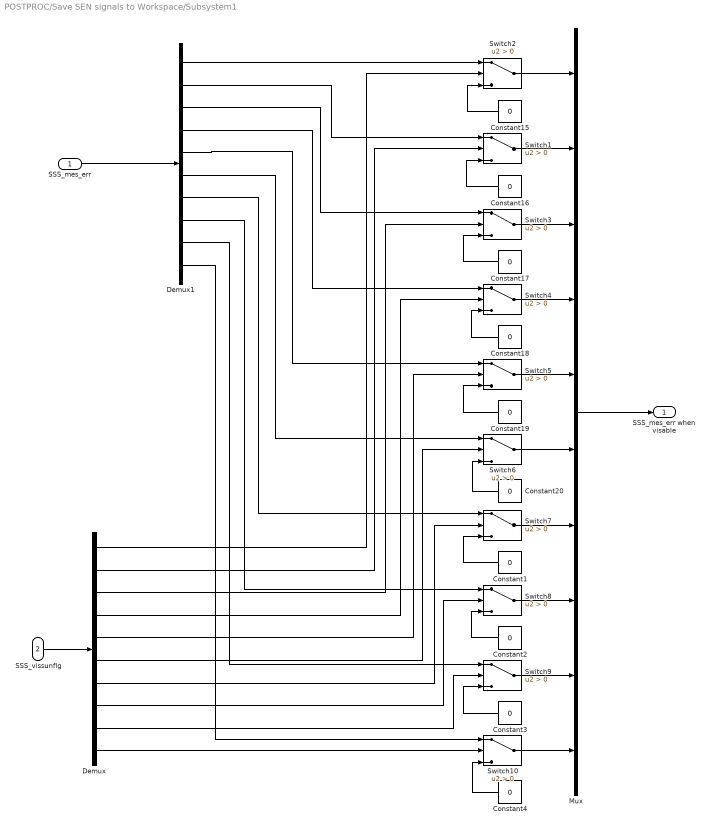
== system POSTPROC/Save SEN signals to Workspace/Subsystem1 ==
  SSS_mes_err : Inport
  SSS_vissunflg : Inport  Port=2
  Constant{1..4,15..20} (10 alike) : Constant  Value=0
  Demux : Demux  Outputs=10
  Demux1 : Demux  Outputs=10
  Mux : Mux  Inputs=10
  Switch{1..10} (10 alike) : Switch  Criteria=u2 > Threshold
  SSS_mes_err when visable : Outport
  wires:
  Demux1/8 -> Switch8/1
  Demux1/7 -> Switch7/1
  Constant4/1 -> Switch10/3
  Constant3/1 -> Switch9/3
  Demux/7 -> Switch7/2
  Switch10/1 -> Mux/10
  Demux/8 -> Switch8/2
  Demux1/9 -> Switch9/1
  Demux1/10 -> Switch10/1
  Constant1/1 -> Switch7/3
  Demux/9 -> Switch9/2
  Constant2/1 -> Switch8/3
  Switch7/1 -> Mux/7
  Switch9/1 -> Mux/9
  Demux/10 -> Switch10/2
  Switch8/1 -> Mux/8
  Constant20/1 -> Switch6/3
  Switch2/1 -> Mux/1
  Constant19/1 -> Switch5/3
  Mux/1 -> SSS_mes_err when visable/1
  Demux/3 -> Switch3/2
  Demux/2 -> Switch1/2
  Switch6/1 -> Mux/6
  Demux1/2 -> Switch1/1
  Demux/4 -> Switch4/2
  Demux1/5 -> Switch5/1
  Demux1/6 -> Switch6/1
  Constant16/1 -> Switch1/3
  Demux1/3 -> Switch3/1
  SSS_mes_err/1 -> Demux1/1
  Demux/1 -> Switch2/2
  Demux1/4 -> Switch4/1
  Constant17/1 -> Switch3/3
  Demux/5 -> Switch5/2
  Constant18/1 -> Switch4/3
  Switch1/1 -> Mux/2
  Demux1/1 -> Switch2/1
  Switch3/1 -> Mux/3
  Switch5/1 -> Mux/5
  Demux/6 -> Switch6/2
  Switch4/1 -> Mux/4
  SSS_vissunflg/1 -> Demux/1
  Constant15/1 -> Switch2/3

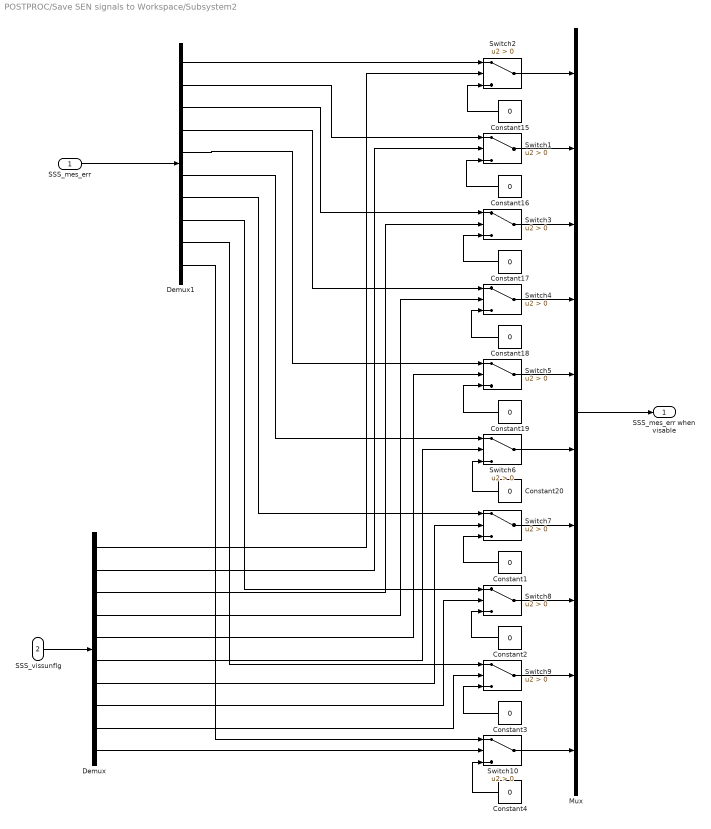
== system POSTPROC/Save SEN signals to Workspace/Subsystem2 ==
  SSS_mes_err : Inport
  SSS_vissunflg : Inport  Port=2
  Constant{1..4,15..20} (10 alike) : Constant  Value=0
  Demux : Demux  Outputs=10
  Demux1 : Demux  Outputs=10
  Mux : Mux  Inputs=10
  Switch{1..10} (10 alike) : Switch  Criteria=u2 > Threshold
  SSS_mes_err when visable : Outport
  wires:
  Constant15/1 -> Switch2/3
  SSS_vissunflg/1 -> Demux/1
  Switch4/1 -> Mux/4
  Demux/6 -> Switch6/2
  Switch5/1 -> Mux/5
  Switch3/1 -> Mux/3
  Demux1/1 -> Switch2/1
  Switch1/1 -> Mux/2
  Constant18/1 -> Switch4/3
  Demux/5 -> Switch5/2
  Constant17/1 -> Switch3/3
  Demux1/4 -> Switch4/1
  Demux/1 -> Switch2/2
  SSS_mes_err/1 -> Demux1/1
  Demux1/3 -> Switch3/1
  Constant16/1 -> Switch1/3
  Demux1/6 -> Switch6/1
  Demux1/5 -> Switch5/1
  Demux/4 -> Switch4/2
  Demux1/2 -> Switch1/1
  Switch6/1 -> Mux/6
  Demux/2 -> Switch1/2
  Demux/3 -> Switch3/2
  Mux/1 -> SSS_mes_err when visable/1
  Constant19/1 -> Switch5/3
  Switch2/1 -> Mux/1
  Constant20/1 -> Switch6/3
  Switch8/1 -> Mux/8
  Demux/10 -> Switch10/2
  Switch9/1 -> Mux/9
  Switch7/1 -> Mux/7
  Constant2/1 -> Switch8/3
  Demux/9 -> Switch9/2
  Constant1/1 -> Switch7/3
  Demux1/10 -> Switch10/1
  Demux1/9 -> Switch9/1
  Demux/8 -> Switch8/2
  Switch10/1 -> Mux/10
  Demux/7 -> Switch7/2
  Constant3/1 -> Switch9/3
  Constant4/1 -> Switch10/3
  Demux1/7 -> Switch7/1
  Demux1/8 -> Switch8/1

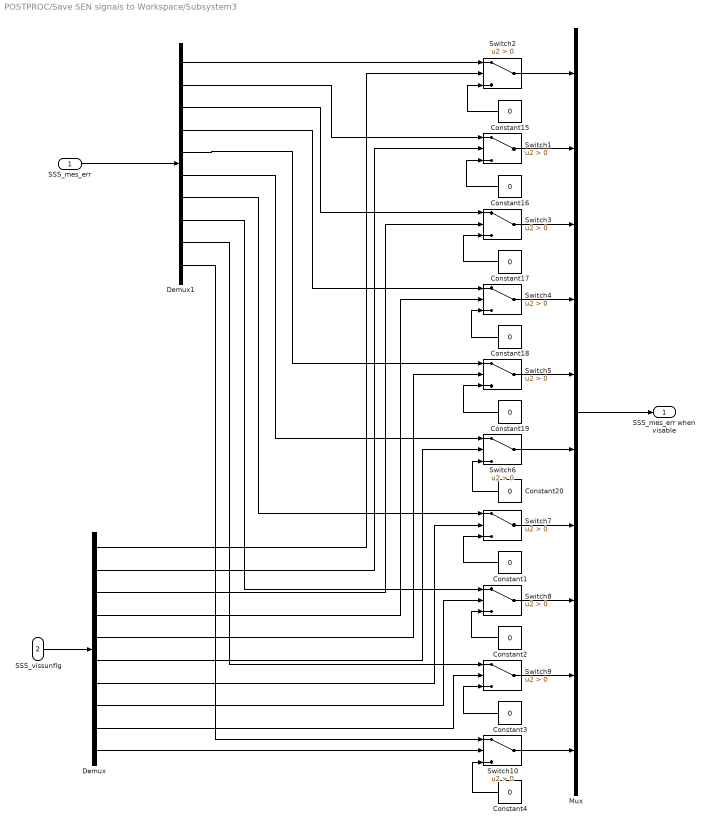
== system POSTPROC/Save SEN signals to Workspace/Subsystem3 ==
  SSS_mes_err : Inport
  SSS_vissunflg : Inport  Port=2
  Constant{1..4,15..20} (10 alike) : Constant  Value=0
  Demux : Demux  Outputs=10
  Demux1 : Demux  Outputs=10
  Mux : Mux  Inputs=10
  Switch{1..10} (10 alike) : Switch  Criteria=u2 > Threshold
  SSS_mes_err when visable : Outport
  wires:
  Constant15/1 -> Switch2/3
  SSS_vissunflg/1 -> Demux/1
  Switch4/1 -> Mux/4
  Demux/6 -> Switch6/2
  Switch5/1 -> Mux/5
  Switch3/1 -> Mux/3
  Demux1/1 -> Switch2/1
  Switch1/1 -> Mux/2
  Constant18/1 -> Switch4/3
  Demux/5 -> Switch5/2
  Constant17/1 -> Switch3/3
  Demux1/4 -> Switch4/1
  Demux/1 -> Switch2/2
  SSS_mes_err/1 -> Demux1/1
  Demux1/3 -> Switch3/1
  Constant16/1 -> Switch1/3
  Demux1/6 -> Switch6/1
  Demux1/5 -> Switch5/1
  Demux/4 -> Switch4/2
  Demux1/2 -> Switch1/1
  Switch6/1 -> Mux/6
  Demux/2 -> Switch1/2
  Demux/3 -> Switch3/2
  Mux/1 -> SSS_mes_err when visable/1
  Constant19/1 -> Switch5/3
  Switch2/1 -> Mux/1
  Constant20/1 -> Switch6/3
  Switch8/1 -> Mux/8
  Demux/10 -> Switch10/2
  Switch9/1 -> Mux/9
  Switch7/1 -> Mux/7
  Constant2/1 -> Switch8/3
  Demux/9 -> Switch9/2
  Constant1/1 -> Switch7/3
  Demux1/10 -> Switch10/1
  Demux1/9 -> Switch9/1
  Demux/8 -> Switch8/2
  Switch10/1 -> Mux/10
  Demux/7 -> Switch7/2
  Constant3/1 -> Switch9/3
  Constant4/1 -> Switch10/3
  Demux1/7 -> Switch7/1
  Demux1/8 -> Switch8/1

== matlab function Save SEN signals to Workspace/MATLAB Function ==
  data: SCsolarflux input double; ADCcount input double; current output double; ADCmaxcurrent input double; adcbits input double; am0 input double; currentpermsq input double; cellarea input double; maxExpectedcurrent output double; maxExpectedcurrent_SFcorrected output double; angle output double; angle_SFcorrected output double
function ...
    [current,                   ...
    maxExpectedcurrent,                 ...
    maxExpectedcurrent_SFcorrected,  ...
    angle,                      ...
    angle_SFcorrected           ...
    ]= fcn(                     ...
    SCsolarflux,                ...
    ADCcount,                   ...
    ADCmaxcurrent,              ...
    adcbits,                    ...
    am0, currentpermsq, cellarea)
  %#codegen
  % determine measured current
  lsb2current = ADCmaxcurrent/2^adcbits;
  current     = ADCcount.* lsb2current;
  
  % figure out maximum expected currents
  maxExpectedcurrent  = currentpermsq*cellarea;
  maxExpectedcurrent_SFcorrected  = SCsolarflux/am0*maxExpectedcurrent;
  
  % compute angle from measured current and max expected currents
  
  
  cosangle = current./maxExpectedcurrent;
  cosangle_corrected = current./maxExpectedcurrent_SFcorrected;
  
  for i=1:1:10
    cosangle(i)= min(cosangle(i),1);
    cosangle(i)= max(cosangle(i),0);
    
    cosangle_corrected(i)= min(cosangle_corrected(i),1);
    cosangle_corrected(i)= max(cosangle_corrected(i),0);
    
  end
  
  
  angle    = acos(cosangle);
  angle_SFcorrected =  acos(cosangle_corrected);
  
  
end
